simulink subsystem "CheckOutput"  (R2021a)
settings: Solver=VariableStepAuto  StartTime=0.0  StopTime=10.0  RelTol=1e-3
undefined symbols (not defined in the file): ErrCodeOut, NoErr, RangeLwOut, RangeUpOut
libraries: simulink x1
settings Model: Creator=zurnmar  LastModifiedBy=zurnmar

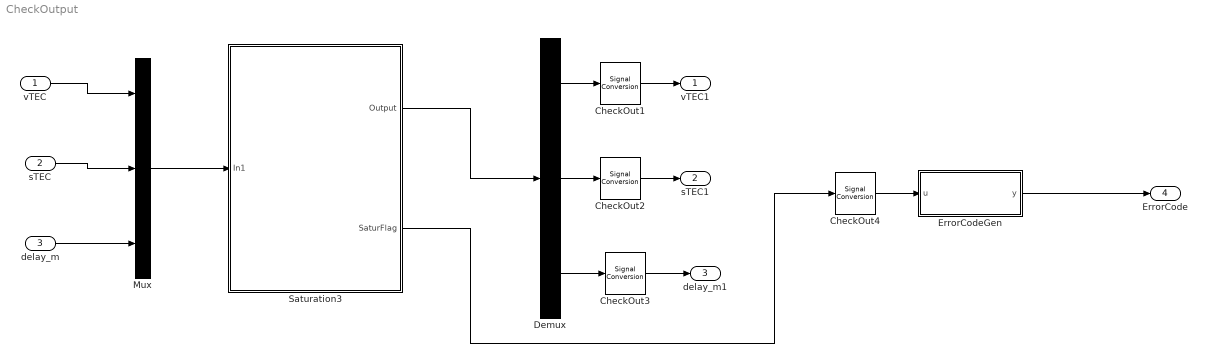
== system CheckOutput ==
  vTEC : Inport
  sTEC : Inport  Port=2
  delay_m : Inport  Port=3
  CheckOut{1..4} (4 alike) : SignalConversion  OverrideOpt=off
  Demux : Demux  Outputs=3
  ErrorCodeGen : Subsystem
  Mux : Mux  Inputs=3
  Saturation3 : Subsystem  TreatAsAtomicUnit=on
      settings: RTWFcnNameOpts=Use subsystem name
  vTEC1 : Outport
  sTEC1 : Outport  Port=2
  delay_m1 : Outport  Port=3
  ErrorCode : Outport  Port=4
  wires:
  ErrorCodeGen/1(y) -> ErrorCode/1
  vTEC/1 -> Mux/1
  sTEC/1 -> Mux/2
  delay_m/1 -> Mux/3
  Mux/1 -> Saturation3/1(In1)
  Demux/3 -> CheckOut3/1
  Demux/1 -> CheckOut1/1
  Demux/2 -> CheckOut2/1
  Saturation3/1(Output) -> Demux/1
  Saturation3/2(SaturFlag) -> CheckOut4/1
  CheckOut1/1 -> vTEC1/1
  CheckOut2/1 -> sTEC1/1
  CheckOut3/1 -> delay_m1/1
  CheckOut4/1 -> ErrorCodeGen/1(u)

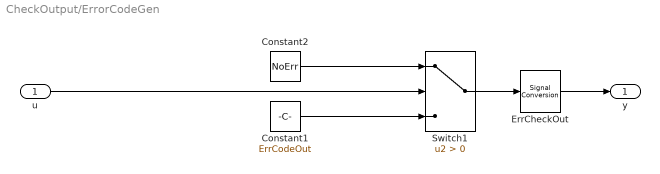
== system CheckOutput/ErrorCodeGen ==
  u : Inport
  Constant1 : Constant  Value=ErrCodeOut  OutDataTypeStr=uint16
  Constant2 : Constant  Value=NoErr
  ErrCheckOut : SignalConversion  OverrideOpt=off
  Switch1 : Switch  Criteria=u2 > Threshold
  y : Outport
  wires:
  ErrCheckOut/1 -> y/1
  Switch1/1 -> ErrCheckOut/1
  Constant1/1 -> Switch1/3
  Constant2/1 -> Switch1/1
  u/1 -> Switch1/2

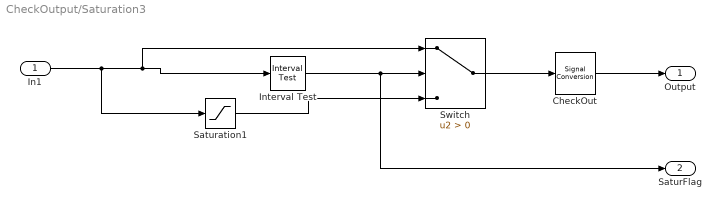
== system CheckOutput/Saturation3 ==
  In1 : Inport
  CheckOut : SignalConversion  OverrideOpt=off
  Interval Test : simulink/Logic and Bit Operations/Interval Test  IntervalClosedRight=on  uplimit=RangeUpOut  IntervalClosedLeft=on  lowlimit=RangeLwOut  OutDataTypeStr=boolean
  Saturation1 : Saturate  UpperLimit=RangeUpOut  LowerLimit=RangeLwOut
  Switch : Switch  Criteria=u2 > Threshold
  Output : Outport
  SaturFlag : Outport  Port=2
  wires:
  CheckOut/1 -> Output/1
  Switch/1 -> CheckOut/1
  In1/1 -> Interval Test/1, Switch/1, Saturation1/1
  Saturation1/1 -> Switch/3
  Interval Test/1 -> Switch/2, SaturFlag/1
